simulink model "JKFF_Model"  (R2023a)
settings: Solver=VariableStepAuto  StartTime=0.0  StopTime=10.0  RelTol=1e-3
libraries: NSA_DEVS_SINKS_ATOMIC x5, NSA_DEVS_SOURCES_ATOMIC x3, NSA_DEVS_DIGITAL_FLIPFLOPS_ATOMIC x1
settings Model: Creator=david  LastModifiedBy=david

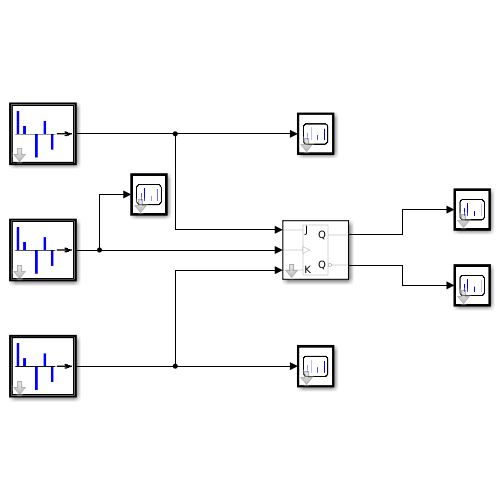
[thumbnail: Simulink's stored preview of the top-level diagram]
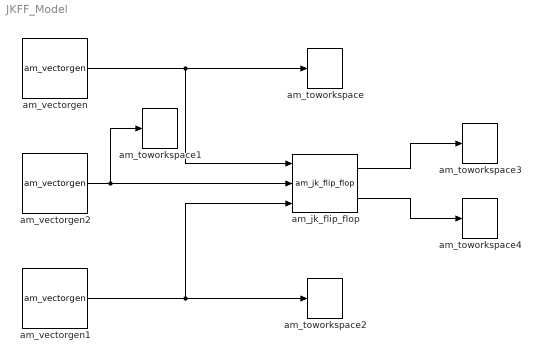
== system JKFF_Model ==
  am_jk_flip_flop : NSA_DEVS_DIGITAL_FLIPFLOPS_ATOMIC/am_jk_flip_flop  q0="\"0\""  tau=[0,1]  debug=0
      settings: SourceProductName=NSA_DEVS
  am_toworkspace : NSA_DEVS_SINKS_ATOMIC/am_toworkspace  varname="\"gen1Out\""  t0=0  format="\"vector\""  tau=[0,5]  debug=0
      settings: SourceProductName=NSA_DEVS
  am_toworkspace1 : NSA_DEVS_SINKS_ATOMIC/am_toworkspace  varname="\"gen3Out\""  t0=0  format="\"vector\""  tau=[0,5]  debug=0
      settings: SourceProductName=NSA_DEVS
  am_toworkspace2 : NSA_DEVS_SINKS_ATOMIC/am_toworkspace  varname="\"gen2Out\""  t0=0  format="\"vector\""  tau=[0,5]  debug=0
      settings: SourceProductName=NSA_DEVS
  am_toworkspace3 : NSA_DEVS_SINKS_ATOMIC/am_toworkspace  varname="\"doutq\""  t0=0  format="\"vector\""  tau=[0,5]  debug=0
      settings: SourceProductName=NSA_DEVS
  am_toworkspace4 : NSA_DEVS_SINKS_ATOMIC/am_toworkspace  varname="\"doutqn\""  t0=0  format="\"vector\""  tau=[0,5]  debug=0
      settings: SourceProductName=NSA_DEVS
  am_vectorgen : NSA_DEVS_SOURCES_ATOMIC/am_vectorgen  tvec="[0, 0.9, 1.1, 4.9,   15, 16.1, 16.3, 16.9, 17.1,   26]"  yvec="[\"0\",   \"1\",   \"0\",   \"1\",    \"0\",    \"1\",    \"0\",    \"1\",    \"0\",    \"0\"]"  tau=[0,1]  debug=0
      settings: SourceProductName=NSA_DEVS
  am_vectorgen1 : NSA_DEVS_SOURCES_ATOMIC/am_vectorgen  tvec="[0, 2.9, 3.1, 4.9,   15, 15.1, 17.3, 17.5, 18.1, 18.5, 20.9, 21.1, 26]"  yvec="[\"0\",   \"1\",   \"0\",   \"1\",    \"0\",    \"0\",    \"1\",    \"0\",    \"1\",    \"0\",    \"1\",    \"0\",  \"0\"]"  tau=[0,1]  debug=0
      settings: SourceProductName=NSA_DEVS
  am_vectorgen2 : NSA_DEVS_SOURCES_ATOMIC/am_vectorgen  tvec=[0, 1, 2, 3, 4, 5, 6, 7, 8, 9, 10, 11, 12, 13, 14, 15, 16, 17, 18]  yvec="[\"0\", \"1\", \"0\", \"1\", \"0\", \"1\", \"0\", \"1\", \"0\", \"1\",  \"0\",  \"1\",  \"0\",  \"1\",  \"0\",  \"1\",  \"0\",  \"1\",  \"0\"]"  tau=[0,1]  debug=0
      settings: SourceProductName=NSA_DEVS
  wires:
  am_vectorgen2/1 -> am_toworkspace1/1, am_jk_flip_flop/2
  am_vectorgen/1 -> am_toworkspace/1, am_jk_flip_flop/1
  am_vectorgen1/1 -> am_toworkspace2/1, am_jk_flip_flop/3
  am_jk_flip_flop/1 -> am_toworkspace3/1
  am_jk_flip_flop/2 -> am_toworkspace4/1
